simulink model "Prediction_3sAdvance_2output"  (R2016b)
settings: Solver=FixedStepAuto  StartTime=0.0  StopTime=length(lat_y)  FixedStep=1  RelTol=1e-3
StopFcn:
  | %%
  | scrsz = get(groot,'ScreenSize');
  | figure('Position',[40 scrsz(4)*0.1 scrsz(3)*0.8 scrsz(4)*0.8])
  | 
  | lng_margin = (max(LOCATIONLongitude(indices))-min(LOCATIONLongitude(indices)))*0.01;
  | lat_margin = (max(LOCATIONLatitude(indices))-min(LOCATIONLatitude(indices)))*0.01;
  | 
  | live_plot_title = ['Pedestrian Path Neural Network Prediction' newline ...
  |     'Green Rectangle:Current Position, Cyan Rectangle:Future Position' newline ...
  |     'blue line:predicted, green line:actual path'];
  | 
  | %occupy space on google map to plot the predicted trajectory
  | annotation('textbox', [0.7 0.9 0.1 0.1],'String', live_plot_title,'EdgeColor', 'k','HorizontalAlignment', 'center','FontWeight','bold');
  | 
  | %plot for acutal pedestrian path
  | subplot(1,2,1);
  | actual_lng = LOCATIONLongitude(indices);
  | actual_lat = LOCATIONLatitude(indices);
  | plot(actual_lng,actual_lat,'g','linewidth',2); hold on;
  | plot_google_map('MapType','satellite');
  | xlim([min(actual_lng)-lng_margin max(actual_lng)+lng_margin]);
  | ylim([min(actual_lat)-lat_margin max(actual_lat)+lat_margin]);
  | title('Actual Pedestrian Path');xlabel('Longitude');ylabel('Latitude');
  | 
  | 
  | predict_y = out_x.signals.values;
  | predict_x = out_y.signals.values;
  | 
  | %convert the predicted path to the latitude and longitude
  | [predict_lat,predict_lng] = utm2ll(predict_y + x_init, predict_x + y_init,zone);
  | subplot(1,2,2);
  | title('Predicted Pedestrian Path');xlabel('Longitude');ylabel('Latitude');
  | lat_lim = [min(predict_lat) min(predict_lat) max(predict_lat) max(predict_lat)];
  | long_lim = [max(predict_lng) min(predict_lng) min(predict_lng) max(predict_lng)];
  | scatter(long_lim, lat_lim);
  | plot_google_map('MapType','satellite');
  | xlim([min(predict_lng)-lng_margin max(predict_lng)+lng_margin]);
  | ylim([min(predict_lat)-lat_margin max(predict_lat)+lat_margin]);
  | for(i=1:1:length(actual_lat))
  |     plot(actual_lng(i),actual_lat(i),'gs','MarkerSize',10);hold on;
  |     plot(predict_lng(i),predict_lat(i),'bs','MarkerSize',10);hold on;
  | 
  |     RectPosCurr = [actual_lng(i)-lng_margin*2 actual_lat(i)-lat_margin*2 lng_margin*4 lat_margin*4];
  |     RectPosFuture = [predict_lng(i)-lng_margin*2 predict_lat(i)-lat_margin*2 lng_margin*4 lat_margin*4];
  |     showCurr = rectangle('Position',RectPosCurr,'FaceColor','g','Visible','on');
  |     showFuture = rectangle('Position',RectPosFuture,'FaceColor','c','Visible','on');
  |     pause(0.01/2);
  | 
  |     set(showCurr,'Visible','off');
  |     set(showFuture,'Visible','off');
  |     pause(0.01/2);
  | end
  | 
  | 
  | save('TestData_NNPred_3s.mat','indices','LOCATIONLatitude','LOCATIONLongitude','predict_lat','predict_lng');
values from neighbouring files (symbols this model uses):
  indices = [20 21 22 23 24 25 26 27 28 29 30 31 ... (1110 elements, 1110x1)]    [Circle.mat]    (also in DoubleEllipse.mat = [57 58 59 60 61 62 63 64 65 66 67 68 ... (2382 elements, 238; GPS_Path_Prediction.m = find(~isempty(orientation_temp)&~isnan(orientation_temp)); Rectangle.mat = [51 52 53 54 55 56 57 58 59 60 61 62 ... (1700 elements, 170; special_filter.m = find(variance<=var_threshold & abs(magnitude) <= mag_thresho)
  LOCATIONLatitude = [42.32249 42.32249 42.32249 42.32249 42.32249 42.32249 42.32249 42.32249 42.32249 42.32249 42.32249 42.32249 ... (1135 elements, 1135x1)]    [Circle.mat]    (also in DoubleEllipse.mat = [42.322384 42.322384 42.322384 42.322384 42.322384 42.322384; Rectangle.mat = [42.323025 42.323025 42.323025 42.323025 42.323025 42.323025)
  LOCATIONLongitude = [-83.479965 -83.479965 -83.479965 -83.479965 -83.479965 -83.479965 -83.479965 -83.479965 -83.479965 -83.479965 -83.479965 -83.479965 ... (1135 elements, 1135x1)]    [Circle.mat]    (also in DoubleEllipse.mat = [-83.47919 -83.47919 -83.47919 -83.47919 -83.47919 -83.47919; Rectangle.mat = [-83.47979 -83.47979 -83.47979 -83.47979 -83.47979 -83.47979)
libraries: neural x17
(part 1 of 2)
settings Model: Creator=divye  LastModifiedBy=divye

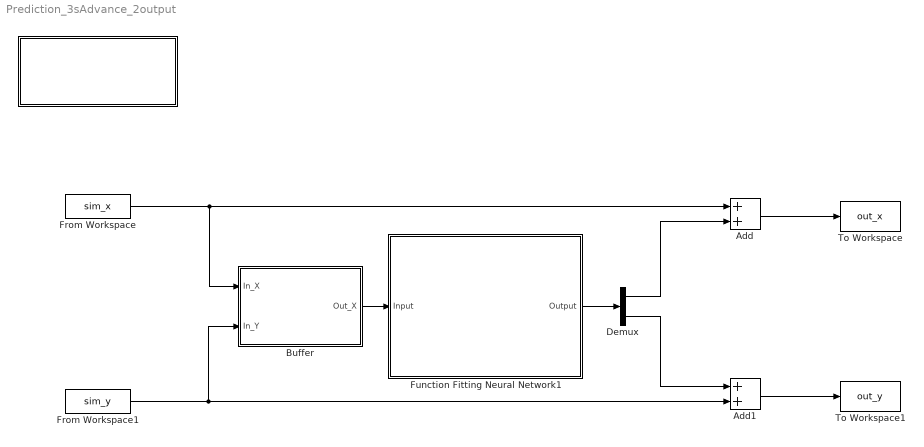
== system Prediction_3sAdvance_2output ==
  " " : Subsystem
      settings: OpenFcn=|
      | %%
      | %receive the user input for the measurement file
      | clear all;close all; %#ok<CLALL>
      | [measurement_file, measurement_file_path] = uigetfile({'*.mat'},'Measurement File Selector');
      | filename = strcat(measurement_file_path,measurement_file);
      | load(filename);
      | t=0:1:length(lng_x)-1;
      | sim_x = [t' lng_x];
      | sim_y = [t' lat_y];
      mask Display: disp(['Import' newline 'Data Set'])
  Add : Sum
  Add1 : Sum
  Buffer : Subsystem
  Demux : Demux  Outputs=2
  From Workspace : FromWorkspace  VariableName=sim_x  SampleTime=1
  From Workspace1 : FromWorkspace  VariableName=sim_y  SampleTime=1
  Function Fitting Neural Network1 : Subsystem
      mask help: Function Fitting Neural Network
      mask Display: e = 0.06;c1 = [120 150 230]/255;c2 = ([120 150 230]+0)/383;c3 = ([120 150 230]+128)/383;patch([0 1 1 0],[0 0 1 1],c1);patch([0 1 1 1-e 1-e 0+e],[0 0 1 1-e 0+e 0+e],c2);patch([0 0 1 1-e 0+e 0+e],[0 1 1 1-e 1-e 0+e],c3);plot([0 1 1 0 0],[0 0 1 1 0]);fprintf('NNET');port_label('input',1,' Input');port_label('output',1,'Output ');
  To Workspace : ToWorkspace  VariableName=out_x  SaveFormat=Structure With Time  SampleTime=-1
  To Workspace1 : ToWorkspace  VariableName=out_y  SaveFormat=Structure With Time  SampleTime=-1
  wires:
  Buffer/1(Out_X) -> Function Fitting Neural Network1/1(Input)
  Function Fitting Neural Network1/1(Output) -> Demux/1
  From Workspace/1 -> Buffer/1(In_X), Add/1
  Demux/1 -> Add/2
  Add/1 -> To Workspace/1
  Demux/2 -> Add1/1
  From Workspace1/1 -> Buffer/2(In_Y), Add1/2
  Add1/1 -> To Workspace1/1

== system Prediction_3sAdvance_2output/  ==

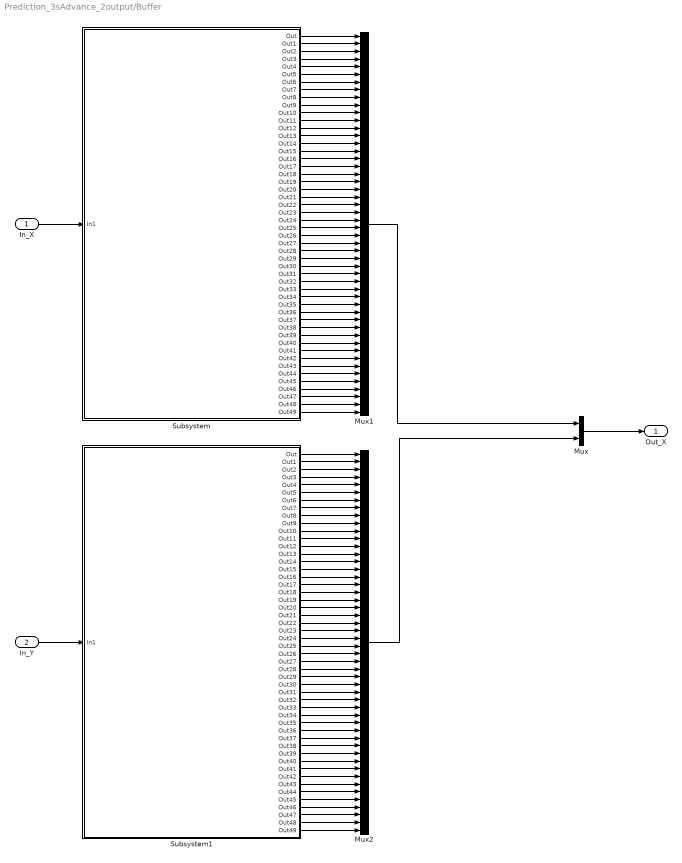
== system Prediction_3sAdvance_2output/Buffer ==
  In_X : Inport
  In_Y : Inport  Port=2
  Mux : Mux  Inputs=2
  Mux1 : Mux  Inputs=50
  Mux2 : Mux  Inputs=50
  Subsystem : Subsystem
  Subsystem1 : Subsystem
  Out_X : Outport
  wires:
  Mux1/1 -> Mux/1
  Subsystem1/46(Out45) -> Mux2/46
  Subsystem1/20(Out19) -> Mux2/20
  Subsystem1/38(Out37) -> Mux2/38
  Subsystem1/21(Out20) -> Mux2/21
  Subsystem1/42(Out41) -> Mux2/42
  Subsystem1/47(Out46) -> Mux2/47
  Subsystem1/22(Out21) -> Mux2/22
  Subsystem1/5(Out4) -> Mux2/5
  In_Y/1 -> Subsystem1/1(In1)
  Subsystem1/43(Out42) -> Mux2/43
  Subsystem1/11(Out10) -> Mux2/11
  In_X/1 -> Subsystem/1(In1)
  Subsystem1/19(Out18) -> Mux2/19
  Subsystem1/23(Out22) -> Mux2/23
  Subsystem1/17(Out16) -> Mux2/17
  Subsystem1/1(Out) -> Mux2/1
  Subsystem1/25(Out24) -> Mux2/25
  Subsystem1/44(Out43) -> Mux2/44
  Subsystem1/37(Out36) -> Mux2/37
  Subsystem1/39(Out38) -> Mux2/39
  Mux2/1 -> Mux/2
  Subsystem1/45(Out44) -> Mux2/45
  Subsystem1/41(Out40) -> Mux2/41
  Subsystem1/14(Out13) -> Mux2/14
  Subsystem1/24(Out23) -> Mux2/24
  Subsystem1/40(Out39) -> Mux2/40
  Subsystem/28(Out27) -> Mux1/28
  Subsystem/48(Out47) -> Mux1/48
  Subsystem/29(Out28) -> Mux1/29
  Subsystem/27(Out26) -> Mux1/27
  Subsystem/34(Out33) -> Mux1/34
  Subsystem/32(Out31) -> Mux1/32
  Subsystem/33(Out32) -> Mux1/33
  Subsystem/30(Out29) -> Mux1/30
  Subsystem/36(Out35) -> Mux1/36
  Subsystem/26(Out25) -> Mux1/26
  Subsystem/49(Out48) -> Mux1/49
  Subsystem/50(Out49) -> Mux1/50
  Subsystem/31(Out30) -> Mux1/31
  Subsystem/3(Out2) -> Mux1/3
  Subsystem/35(Out34) -> Mux1/35
  Subsystem/2(Out1) -> Mux1/2
  Subsystem/22(Out21) -> Mux1/22
  Subsystem/15(Out14) -> Mux1/15
  Subsystem/19(Out18) -> Mux1/19
  Subsystem/24(Out23) -> Mux1/24
  Subsystem/20(Out19) -> Mux1/20
  Subsystem/4(Out3) -> Mux1/4
  Subsystem/9(Out8) -> Mux1/9
  Subsystem/13(Out12) -> Mux1/13
  Subsystem/12(Out11) -> Mux1/12
  Subsystem/10(Out9) -> Mux1/10
  Subsystem/16(Out15) -> Mux1/16
  Subsystem/6(Out5) -> Mux1/6
  Subsystem/7(Out6) -> Mux1/7
  Subsystem/8(Out7) -> Mux1/8
  Subsystem/18(Out17) -> Mux1/18
  Subsystem/17(Out16) -> Mux1/17
  Subsystem/25(Out24) -> Mux1/25
  Subsystem/23(Out22) -> Mux1/23
  Subsystem/21(Out20) -> Mux1/21
  Subsystem/14(Out13) -> Mux1/14
  Subsystem/43(Out42) -> Mux1/43
  Subsystem/42(Out41) -> Mux1/42
  Subsystem/41(Out40) -> Mux1/41
  Subsystem/46(Out45) -> Mux1/46
  Subsystem/37(Out36) -> Mux1/37
  Subsystem/45(Out44) -> Mux1/45
  Subsystem/40(Out39) -> Mux1/40
  Subsystem/47(Out46) -> Mux1/47
  Subsystem/5(Out4) -> Mux1/5
  Subsystem/44(Out43) -> Mux1/44
  Subsystem/38(Out37) -> Mux1/38
  Subsystem/39(Out38) -> Mux1/39
  Subsystem/11(Out10) -> Mux1/11
  Subsystem/1(Out) -> Mux1/1
  Subsystem1/49(Out48) -> Mux2/49
  Subsystem1/48(Out47) -> Mux2/48
  Subsystem1/50(Out49) -> Mux2/50
  Subsystem1/28(Out27) -> Mux2/28
  Subsystem1/29(Out28) -> Mux2/29
  Subsystem1/33(Out32) -> Mux2/33
  Subsystem1/4(Out3) -> Mux2/4
  Subsystem1/2(Out1) -> Mux2/2
  Subsystem1/9(Out8) -> Mux2/9
  Subsystem1/30(Out29) -> Mux2/30
  Subsystem1/31(Out30) -> Mux2/31
  Subsystem1/34(Out33) -> Mux2/34
  Subsystem1/32(Out31) -> Mux2/32
  Subsystem1/13(Out12) -> Mux2/13
  Subsystem1/10(Out9) -> Mux2/10
  Subsystem1/15(Out14) -> Mux2/15
  Subsystem1/26(Out25) -> Mux2/26
  Subsystem1/27(Out26) -> Mux2/27
  Subsystem1/8(Out7) -> Mux2/8
  Subsystem1/18(Out17) -> Mux2/18
  Subsystem1/16(Out15) -> Mux2/16
  Subsystem1/36(Out35) -> Mux2/36
  Subsystem1/12(Out11) -> Mux2/12
  Subsystem1/35(Out34) -> Mux2/35
  Subsystem1/7(Out6) -> Mux2/7
  Subsystem1/3(Out2) -> Mux2/3
  Subsystem1/6(Out5) -> Mux2/6
  Mux/1 -> Out_X/1

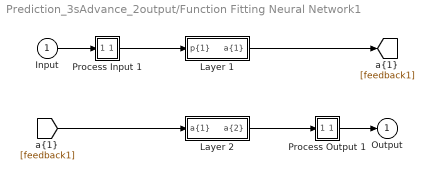
== system Prediction_3sAdvance_2output/Function Fitting Neural Network1 ==
  Input : Inport  PortDimensions=100
      mask Display: e = 0.06;c1 = [120 230 180]/255;c2 = ([120 230 180]+0)/(256+128);c3 = ([120 230 180]+128)/(256+128);patch([0 1 1 0],[0 0 1 1],c1);patch([0 1 1 1-e 1-e 0+e],[0 0 1 1-e 0+e 0+e],c2);patch([0 0 1 1-e 0+e 0+e],[0 1 1 1-e 1-e 0+e],c3);plot([0 1 1 0 0],[0 0 1 1 0]);
  Layer 1 : Subsystem
      mask Display: e = 0.06;c1 = [120 150 230]/255;c2 = ([120 150 230]+0)/383;c3 = ([120 150 230]+128)/383;patch([0 1 1 0],[0 0 1 1],c1);patch([0 1 1 1-e 1-e 0+e],[0 0 1 1-e 0+e 0+e],c2);patch([0 0 1 1-e 0+e 0+e],[0 1 1 1-e 1-e 0+e],c3);plot([0 1 1 0 0],[0 0 1 1 0]);
  Layer 2 : Subsystem
      mask Display: e = 0.06;c1 = [120 150 230]/255;c2 = ([120 150 230]+0)/383;c3 = ([120 150 230]+128)/383;patch([0 1 1 0],[0 0 1 1],c1);patch([0 1 1 1-e 1-e 0+e],[0 0 1 1-e 0+e 0+e],c2);patch([0 0 1 1-e 0+e 0+e],[0 1 1 1-e 1-e 0+e],c3);plot([0 1 1 0 0],[0 0 1 1 0]);
  Process Input 1 : Subsystem
      mask Display: e = 0.06;c1 = [120 150 230]/255;c2 = ([120 150 230]+0)/383;c3 = ([120 150 230]+128)/383;patch([0 1 1 0],[0 0 1 1],c1);patch([0 1 1 1-e 1-e 0+e],[0 0 1 1-e 0+e 0+e],c2);patch([0 0 1 1-e 0+e 0+e],[0 1 1 1-e 1-e 0+e],c3);plot([0 1 1 0 0],[0 0 1 1 0]);
  Process Output 1 : Subsystem
      mask Display: e = 0.06;c1 = [120 150 230]/255;c2 = ([120 150 230]+0)/383;c3 = ([120 150 230]+128)/383;patch([0 1 1 0],[0 0 1 1],c1);patch([0 1 1 1-e 1-e 0+e],[0 0 1 1-e 0+e 0+e],c2);patch([0 0 1 1-e 0+e 0+e],[0 1 1 1-e 1-e 0+e],c3);plot([0 1 1 0 0],[0 0 1 1 0]);
  Output : Outport  InitialOutput=[0;0]
      mask Display: e = 0.06;c1 = [120 230 180]/255;c2 = ([120 230 180]+0)/(256+128);c3 = ([120 230 180]+128)/(256+128);patch([0 1 1 0],[0 0 1 1],c1);patch([0 1 1 1-e 1-e 0+e],[0 0 1 1-e 0+e 0+e],c2);patch([0 0 1 1-e 0+e 0+e],[0 1 1 1-e 1-e 0+e],c3);plot([0 1 1 0 0],[0 0 1 1 0]);
  wires:
  Input/1 -> Process Input 1/1(x)
  Process Output 1/1(y) -> Output/1
  Process Input 1/1(p) -> Layer 1/1("p{1}")
  Layer 1/1("a{1}") -> [feedback1]
  [feedback1] -> Layer 2/1("a{1} ")
  Layer 2/1("a{2}") -> Process Output 1/1(a)

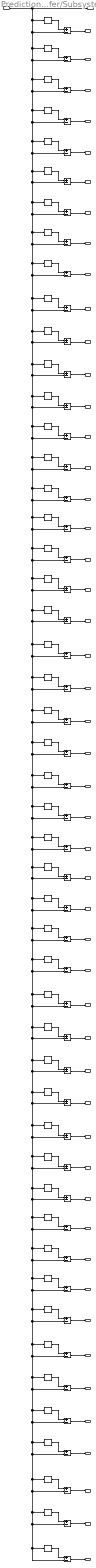
== system Prediction_3sAdvance_2output/Buffer/Subsystem ==
  In1 : Inport
  Delay : Delay  DelayLength=1
  Delay1 : Delay
  Delay10 : Delay  DelayLength=11
  Delay11 : Delay  DelayLength=12
  Delay12 : Delay  DelayLength=13
  Delay13 : Delay  DelayLength=22
  Delay14 : Delay  DelayLength=23
  Delay15 : Delay  DelayLength=24
  Delay16 : Delay  DelayLength=14
  Delay17 : Delay  DelayLength=15
  Delay18 : Delay  DelayLength=16
  Delay19 : Delay  DelayLength=17
  Delay2 : Delay  DelayLength=3
  Delay20 : Delay  DelayLength=18
  Delay21 : Delay  DelayLength=19
  Delay22 : Delay  DelayLength=20
  Delay23 : Delay  DelayLength=21
  Delay24 : Delay  DelayLength=33
  Delay25 : Delay  DelayLength=34
  Delay26 : Delay  DelayLength=35
  Delay27 : Delay  DelayLength=25
  Delay28 : Delay  DelayLength=26
  Delay29 : Delay  DelayLength=27
  Delay3 : Delay  DelayLength=4
  Delay30 : Delay  DelayLength=28
  Delay31 : Delay  DelayLength=29
  Delay32 : Delay  DelayLength=30
  Delay33 : Delay  DelayLength=31
  Delay34 : Delay  DelayLength=32
  Delay35 : Delay  DelayLength=44
  Delay36 : Delay  DelayLength=45
  Delay37 : Delay  DelayLength=46
  Delay38 : Delay  DelayLength=36
  Delay39 : Delay  DelayLength=37
  Delay4 : Delay  DelayLength=5
  Delay40 : Delay  DelayLength=38
  Delay41 : Delay  DelayLength=39
  Delay42 : Delay  DelayLength=40
  Delay43 : Delay  DelayLength=41
  Delay44 : Delay  DelayLength=42
  Delay45 : Delay  DelayLength=43
  Delay46 : Delay  DelayLength=47
  Delay47 : Delay  DelayLength=48
  Delay48 : Delay  DelayLength=49
  Delay5 : Delay  DelayLength=6
  Delay6 : Delay  DelayLength=7
  Delay7 : Delay  DelayLength=8
  Delay8 : Delay  DelayLength=9
  Delay9 : Delay  DelayLength=10
  Subtract{,1..48} (49 alike) : Sum  Inputs=+-
  Out : Outport
  Out1 : Outport  Port=2
  Out2 : Outport  Port=3
  Out3 : Outport  Port=4
  Out4 : Outport  Port=5
  Out5 : Outport  Port=6
  Out6 : Outport  Port=7
  Out7 : Outport  Port=8
  Out8 : Outport  Port=9
  Out9 : Outport  Port=10
  Out10 : Outport  Port=11
  Out11 : Outport  Port=12
  Out12 : Outport  Port=13
  Out13 : Outport  Port=14
  Out14 : Outport  Port=15
  Out15 : Outport  Port=16
  Out16 : Outport  Port=17
  Out17 : Outport  Port=18
  Out18 : Outport  Port=19
  Out19 : Outport  Port=20
  Out20 : Outport  Port=21
  Out21 : Outport  Port=22
  Out22 : Outport  Port=23
  Out23 : Outport  Port=24
  Out24 : Outport  Port=25
  Out25 : Outport  Port=26
  Out26 : Outport  Port=27
  Out27 : Outport  Port=28
  Out28 : Outport  Port=29
  Out29 : Outport  Port=30
  Out30 : Outport  Port=31
  Out31 : Outport  Port=32
  Out32 : Outport  Port=33
  Out33 : Outport  Port=34
  Out34 : Outport  Port=35
  Out35 : Outport  Port=36
  Out36 : Outport  Port=37
  Out37 : Outport  Port=38
  Out38 : Outport  Port=39
  Out39 : Outport  Port=40
  Out40 : Outport  Port=41
  Out41 : Outport  Port=42
  Out42 : Outport  Port=43
  Out43 : Outport  Port=44
  Out44 : Outport  Port=45
  Out45 : Outport  Port=46
  Out46 : Outport  Port=47
  Out47 : Outport  Port=48
  Out48 : Outport  Port=49
  Out49 : Outport  Port=50
  wires:
  Delay/1 -> Subtract/1
  Subtract/1 -> Out1/1
  Delay1/1 -> Subtract1/1
  Subtract1/1 -> Out2/1
  Delay2/1 -> Subtract2/1
  Subtract2/1 -> Out3/1
  Delay3/1 -> Subtract3/1
  Subtract3/1 -> Out4/1
  Delay4/1 -> Subtract4/1
  Subtract4/1 -> Out5/1
  Delay5/1 -> Subtract5/1
  Subtract5/1 -> Out6/1
  Delay6/1 -> Subtract6/1
  Subtract6/1 -> Out7/1
  Delay7/1 -> Subtract7/1
  Subtract7/1 -> Out8/1
  Delay8/1 -> Subtract8/1
  Subtract8/1 -> Out9/1
  Delay9/1 -> Subtract9/1
  Subtract9/1 -> Out10/1
  Delay10/1 -> Subtract10/1
  Subtract10/1 -> Out11/1
  Delay11/1 -> Subtract11/1
  Subtract11/1 -> Out12/1
  Delay12/1 -> Subtract12/1
  Subtract12/1 -> Out13/1
  Delay16/1 -> Subtract16/1
  Subtract16/1 -> Out14/1
  Delay17/1 -> Subtract17/1
  Subtract17/1 -> Out15/1
  Delay18/1 -> Subtract18/1
  Subtract18/1 -> Out16/1
  Delay19/1 -> Subtract19/1
  Subtract19/1 -> Out17/1
  Delay20/1 -> Subtract20/1
  Subtract20/1 -> Out18/1
  Delay21/1 -> Subtract21/1
  Subtract21/1 -> Out19/1
  Delay22/1 -> Subtract22/1
  Subtract22/1 -> Out20/1
  Delay23/1 -> Subtract23/1
  Subtract23/1 -> Out21/1
  Delay13/1 -> Subtract13/1
  Subtract13/1 -> Out22/1
  Delay14/1 -> Subtract14/1
  Subtract14/1 -> Out23/1
  Delay15/1 -> Subtract15/1
  Subtract15/1 -> Out24/1
  Delay27/1 -> Subtract27/1
  Subtract27/1 -> Out25/1
  Delay28/1 -> Subtract28/1
  Subtract28/1 -> Out26/1
  Delay29/1 -> Subtract29/1
  Subtract29/1 -> Out27/1
  Delay30/1 -> Subtract30/1
  Subtract30/1 -> Out28/1
  Delay31/1 -> Subtract31/1
  Subtract31/1 -> Out29/1
  Delay32/1 -> Subtract32/1
  Subtract32/1 -> Out30/1
  Delay33/1 -> Subtract33/1
  Subtract33/1 -> Out31/1
  Delay34/1 -> Subtract34/1
  Subtract34/1 -> Out32/1
  Delay24/1 -> Subtract24/1
  Subtract24/1 -> Out33/1
  Delay25/1 -> Subtract25/1
  Subtract25/1 -> Out34/1
  Delay26/1 -> Subtract26/1
  Subtract26/1 -> Out35/1
  Delay38/1 -> Subtract38/1
  Subtract38/1 -> Out36/1
  Delay39/1 -> Subtract39/1
  Subtract39/1 -> Out37/1
  Delay40/1 -> Subtract40/1
  Subtract40/1 -> Out38/1
  Delay41/1 -> Subtract41/1
  Subtract41/1 -> Out39/1
  Delay42/1 -> Subtract42/1
  Subtract42/1 -> Out40/1
  Delay43/1 -> Subtract43/1
  Subtract43/1 -> Out41/1
  Delay44/1 -> Subtract44/1
  Subtract44/1 -> Out42/1
  Delay45/1 -> Subtract45/1
  Subtract45/1 -> Out43/1
  Delay35/1 -> Subtract35/1
  Subtract35/1 -> Out44/1
  Delay36/1 -> Subtract36/1
  Subtract36/1 -> Out45/1
  Delay37/1 -> Subtract37/1
  Subtract37/1 -> Out46/1
  Delay46/1 -> Subtract46/1
  Subtract46/1 -> Out47/1
  Delay47/1 -> Subtract47/1
  Subtract47/1 -> Out48/1
  Delay48/1 -> Subtract48/1
  Subtract48/1 -> Out49/1
  In1/1 -> Out/1, Delay/1, Subtract/2, Delay1/1, Delay2/1, Delay3/1, Delay4/1, Delay5/1, Delay6/1, Delay7/1, Delay8/1, Delay9/1, Delay10/1, Delay11/1, Delay12/1, Delay16/1, Delay17/1, Delay18/1, Delay19/1, Delay20/1, Delay21/1, Delay22/1, Delay23/1, Delay13/1, Delay14/1, Delay15/1, Delay27/1, Delay28/1, Delay29/1, Delay30/1, Delay31/1, Delay32/1, Delay33/1, Delay34/1, Delay24/1, Delay25/1, Delay26/1, Delay38/1, Delay39/1, Delay40/1, Delay41/1, Delay42/1, Delay43/1, Delay44/1, Delay45/1, Delay35/1, Delay36/1, Delay37/1, Delay46/1, Delay47/1, Delay48/1, Subtract48/2, Subtract47/2, Subtract46/2, Subtract37/2, Subtract36/2, Subtract35/2, Subtract45/2, Subtract44/2, Subtract43/2, Subtract42/2, Subtract41/2, Subtract40/2, Subtract39/2, Subtract38/2, Subtract26/2, Subtract25/2, Subtract24/2, Subtract34/2, Subtract33/2, Subtract32/2, Subtract31/2, Subtract30/2, Subtract29/2, Subtract28/2, Subtract27/2, Subtract15/2, Subtract14/2, Subtract13/2, Subtract23/2, Subtract22/2, Subtract21/2, Subtract20/2, Subtract19/2, Subtract18/2, Subtract17/2, Subtract16/2, Subtract12/2, Subtract11/2, Subtract10/2, Subtract9/2, Subtract8/2, Subtract7/2, Subtract6/2, Subtract5/2, Subtract4/2, Subtract3/2, Subtract2/2, Subtract1/2

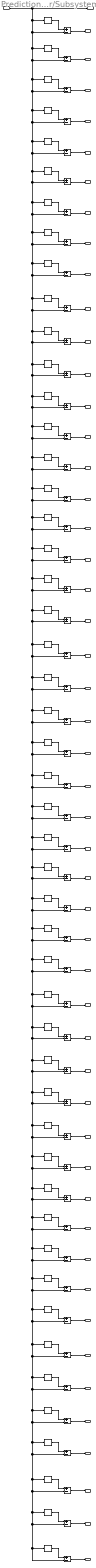
== system Prediction_3sAdvance_2output/Buffer/Subsystem1 ==
  In1 : Inport
  Delay : Delay  DelayLength=1
  Delay1 : Delay
  Delay10 : Delay  DelayLength=11
  Delay11 : Delay  DelayLength=12
  Delay12 : Delay  DelayLength=13
  Delay13 : Delay  DelayLength=22
  Delay14 : Delay  DelayLength=23
  Delay15 : Delay  DelayLength=24
  Delay16 : Delay  DelayLength=14
  Delay17 : Delay  DelayLength=15
  Delay18 : Delay  DelayLength=16
  Delay19 : Delay  DelayLength=17
  Delay2 : Delay  DelayLength=3
  Delay20 : Delay  DelayLength=18
  Delay21 : Delay  DelayLength=19
  Delay22 : Delay  DelayLength=20
  Delay23 : Delay  DelayLength=21
  Delay24 : Delay  DelayLength=33
  Delay25 : Delay  DelayLength=34
  Delay26 : Delay  DelayLength=35
  Delay27 : Delay  DelayLength=25
  Delay28 : Delay  DelayLength=26
  Delay29 : Delay  DelayLength=27
  Delay3 : Delay  DelayLength=4
  Delay30 : Delay  DelayLength=28
  Delay31 : Delay  DelayLength=29
  Delay32 : Delay  DelayLength=30
  Delay33 : Delay  DelayLength=31
  Delay34 : Delay  DelayLength=32
  Delay35 : Delay  DelayLength=44
  Delay36 : Delay  DelayLength=45
  Delay37 : Delay  DelayLength=46
  Delay38 : Delay  DelayLength=36
  Delay39 : Delay  DelayLength=37
  Delay4 : Delay  DelayLength=5
  Delay40 : Delay  DelayLength=38
  Delay41 : Delay  DelayLength=39
  Delay42 : Delay  DelayLength=40
  Delay43 : Delay  DelayLength=41
  Delay44 : Delay  DelayLength=42
  Delay45 : Delay  DelayLength=43
  Delay46 : Delay  DelayLength=47
  Delay47 : Delay  DelayLength=48
  Delay48 : Delay  DelayLength=49
  Delay5 : Delay  DelayLength=6
  Delay6 : Delay  DelayLength=7
  Delay7 : Delay  DelayLength=8
  Delay8 : Delay  DelayLength=9
  Delay9 : Delay  DelayLength=10
  Subtract{,1..48} (49 alike) : Sum  Inputs=+-
  Out : Outport
  Out1 : Outport  Port=2
  Out2 : Outport  Port=3
  Out3 : Outport  Port=4
  Out4 : Outport  Port=5
  Out5 : Outport  Port=6
  Out6 : Outport  Port=7
  Out7 : Outport  Port=8
  Out8 : Outport  Port=9
  Out9 : Outport  Port=10
  Out10 : Outport  Port=11
  Out11 : Outport  Port=12
  Out12 : Outport  Port=13
  Out13 : Outport  Port=14
  Out14 : Outport  Port=15
  Out15 : Outport  Port=16
  Out16 : Outport  Port=17
  Out17 : Outport  Port=18
  Out18 : Outport  Port=19
  Out19 : Outport  Port=20
  Out20 : Outport  Port=21
  Out21 : Outport  Port=22
  Out22 : Outport  Port=23
  Out23 : Outport  Port=24
  Out24 : Outport  Port=25
  Out25 : Outport  Port=26
  Out26 : Outport  Port=27
  Out27 : Outport  Port=28
  Out28 : Outport  Port=29
  Out29 : Outport  Port=30
  Out30 : Outport  Port=31
  Out31 : Outport  Port=32
  Out32 : Outport  Port=33
  Out33 : Outport  Port=34
  Out34 : Outport  Port=35
  Out35 : Outport  Port=36
  Out36 : Outport  Port=37
  Out37 : Outport  Port=38
  Out38 : Outport  Port=39
  Out39 : Outport  Port=40
  Out40 : Outport  Port=41
  Out41 : Outport  Port=42
  Out42 : Outport  Port=43
  Out43 : Outport  Port=44
  Out44 : Outport  Port=45
  Out45 : Outport  Port=46
  Out46 : Outport  Port=47
  Out47 : Outport  Port=48
  Out48 : Outport  Port=49
  Out49 : Outport  Port=50
  wires:
  Delay/1 -> Subtract/1
  Subtract/1 -> Out1/1
  Delay1/1 -> Subtract1/1
  Subtract1/1 -> Out2/1
  Delay2/1 -> Subtract2/1
  Subtract2/1 -> Out3/1
  Delay3/1 -> Subtract3/1
  Subtract3/1 -> Out4/1
  Delay4/1 -> Subtract4/1
  Subtract4/1 -> Out5/1
  Delay5/1 -> Subtract5/1
  Subtract5/1 -> Out6/1
  Delay6/1 -> Subtract6/1
  Subtract6/1 -> Out7/1
  Delay7/1 -> Subtract7/1
  Subtract7/1 -> Out8/1
  Delay8/1 -> Subtract8/1
  Subtract8/1 -> Out9/1
  Delay9/1 -> Subtract9/1
  Subtract9/1 -> Out10/1
  Delay10/1 -> Subtract10/1
  Subtract10/1 -> Out11/1
  Delay11/1 -> Subtract11/1
  Subtract11/1 -> Out12/1
  Delay12/1 -> Subtract12/1
  Subtract12/1 -> Out13/1
  Delay16/1 -> Subtract16/1
  Subtract16/1 -> Out14/1
  Delay17/1 -> Subtract17/1
  Subtract17/1 -> Out15/1
  Delay18/1 -> Subtract18/1
  Subtract18/1 -> Out16/1
  Delay19/1 -> Subtract19/1
  Subtract19/1 -> Out17/1
  Delay20/1 -> Subtract20/1
  Subtract20/1 -> Out18/1
  Delay21/1 -> Subtract21/1
  Subtract21/1 -> Out19/1
  Delay22/1 -> Subtract22/1
  Subtract22/1 -> Out20/1
  Delay23/1 -> Subtract23/1
  Subtract23/1 -> Out21/1
  Delay13/1 -> Subtract13/1
  Subtract13/1 -> Out22/1
  Delay14/1 -> Subtract14/1
  Subtract14/1 -> Out23/1
  Delay15/1 -> Subtract15/1
  Subtract15/1 -> Out24/1
  Delay27/1 -> Subtract27/1
  Subtract27/1 -> Out25/1
  Delay28/1 -> Subtract28/1
  Subtract28/1 -> Out26/1
  Delay29/1 -> Subtract29/1
  Subtract29/1 -> Out27/1
  Delay30/1 -> Subtract30/1
  Subtract30/1 -> Out28/1
  Delay31/1 -> Subtract31/1
  Subtract31/1 -> Out29/1
  Delay32/1 -> Subtract32/1
  Subtract32/1 -> Out30/1
  Delay33/1 -> Subtract33/1
  Subtract33/1 -> Out31/1
  Delay34/1 -> Subtract34/1
  Subtract34/1 -> Out32/1
  Delay24/1 -> Subtract24/1
  Subtract24/1 -> Out33/1
  Delay25/1 -> Subtract25/1
  Subtract25/1 -> Out34/1
  Delay26/1 -> Subtract26/1
  Subtract26/1 -> Out35/1
  Delay38/1 -> Subtract38/1
  Subtract38/1 -> Out36/1
  Delay39/1 -> Subtract39/1
  Subtract39/1 -> Out37/1
  Delay40/1 -> Subtract40/1
  Subtract40/1 -> Out38/1
  Delay41/1 -> Subtract41/1
  Subtract41/1 -> Out39/1
  Delay42/1 -> Subtract42/1
  Subtract42/1 -> Out40/1
  Delay43/1 -> Subtract43/1
  Subtract43/1 -> Out41/1
  Delay44/1 -> Subtract44/1
  Subtract44/1 -> Out42/1
  Delay45/1 -> Subtract45/1
  Subtract45/1 -> Out43/1
  Delay35/1 -> Subtract35/1
  Subtract35/1 -> Out44/1
  Delay36/1 -> Subtract36/1
  Subtract36/1 -> Out45/1
  Delay37/1 -> Subtract37/1
  Subtract37/1 -> Out46/1
  Delay46/1 -> Subtract46/1
  Subtract46/1 -> Out47/1
  Delay47/1 -> Subtract47/1
  Subtract47/1 -> Out48/1
  Delay48/1 -> Subtract48/1
  Subtract48/1 -> Out49/1
  In1/1 -> Out/1, Delay/1, Subtract/2, Delay1/1, Delay2/1, Delay3/1, Delay4/1, Delay5/1, Delay6/1, Delay7/1, Delay8/1, Delay9/1, Delay10/1, Delay11/1, Delay12/1, Delay16/1, Delay17/1, Delay18/1, Delay19/1, Delay20/1, Delay21/1, Delay22/1, Delay23/1, Delay13/1, Delay14/1, Delay15/1, Delay27/1, Delay28/1, Delay29/1, Delay30/1, Delay31/1, Delay32/1, Delay33/1, Delay34/1, Delay24/1, Delay25/1, Delay26/1, Delay38/1, Delay39/1, Delay40/1, Delay41/1, Delay42/1, Delay43/1, Delay44/1, Delay45/1, Delay35/1, Delay36/1, Delay37/1, Delay46/1, Delay47/1, Delay48/1, Subtract48/2, Subtract47/2, Subtract46/2, Subtract37/2, Subtract36/2, Subtract35/2, Subtract45/2, Subtract44/2, Subtract43/2, Subtract42/2, Subtract41/2, Subtract40/2, Subtract39/2, Subtract38/2, Subtract26/2, Subtract25/2, Subtract24/2, Subtract34/2, Subtract33/2, Subtract32/2, Subtract31/2, Subtract30/2, Subtract29/2, Subtract28/2, Subtract27/2, Subtract15/2, Subtract14/2, Subtract13/2, Subtract23/2, Subtract22/2, Subtract21/2, Subtract20/2, Subtract19/2, Subtract18/2, Subtract17/2, Subtract16/2, Subtract12/2, Subtract11/2, Subtract10/2, Subtract9/2, Subtract8/2, Subtract7/2, Subtract6/2, Subtract5/2, Subtract4/2, Subtract3/2, Subtract2/2, Subtract1/2

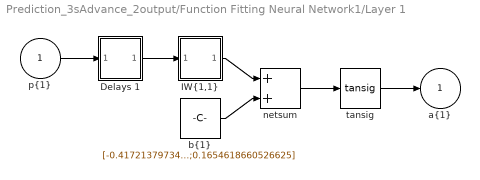
== system Prediction_3sAdvance_2output/Function Fitting Neural Network1/Layer 1 ==
  "p{1}" : Inport  PortDimensions=98
      mask Display: e = 0.06;c1 = [120 230 180]/255;c2 = ([120 230 180]+0)/(256+128);c3 = ([120 230 180]+128)/(256+128);patch([0 1 1 0],[0 0 1 1],c1);patch([0 1 1 1-e 1-e 0+e],[0 0 1 1-e 0+e 0+e],c2);patch([0 0 1 1-e 0+e 0+e],[0 1 1 1-e 1-e 0+e],c3);plot([0 1 1 0 0],[0 0 1 1 0]);
  Delays 1 : Subsystem
      mask Display: e = 0.06;c1 = [120 150 230]/255;c2 = ([120 150 230]+0)/383;c3 = ([120 150 230]+128)/383;patch([0 1 1 0],[0 0 1 1],c1);patch([0 1 1 1-e 1-e 0+e],[0 0 1 1-e 0+e 0+e],c2);patch([0 0 1 1-e 0+e 0+e],[0 1 1 1-e 1-e 0+e],c3);plot([0 1 1 0 0],[0 0 1 1 0]);disp('0');
  "IW{1,1}" : Subsystem
      mask Display: e = 0.06;c1 = [120 150 230]/255;c2 = ([120 150 230]+0)/383;c3 = ([120 150 230]+128)/383;patch([0 1 1 0],[0 0 1 1],c1);patch([0 1 1 1-e 1-e 0+e],[0 0 1 1-e 0+e 0+e],c2);patch([0 0 1 1-e 0+e 0+e],[0 1 1 1-e 1-e 0+e],c3);plot([0 1 1 0 0],[0 0 1 1 0]);disp('W');
  "b{1}" : Constant  Value=[-0.41721379734681036;-0.25154480672700869;0.23985399354268783;0.30750090765798449;-0.47802697511933573;0.040020410928868169;-0.087149329135770795;0.30775217103319574;0.16446617888273593;0.1654618660526625]
      mask Display: e = 0.06;c1 = [120 150 230]/255;c2 = ([120 150 230]+0)/383;c3 = ([120 150 230]+128)/383;patch([0 1 1 0],[0 0 1 1],c1);patch([0 1 1 1-e 1-e 0+e],[0 0 1 1-e 0+e 0+e],c2);patch([0 0 1 1-e 0+e 0+e],[0 1 1 1-e 1-e 0+e],c3);plot([0 1 1 0 0],[0 0 1 1 0]);disp('b');
  netsum : Sum  Inputs=2  SaturateOnIntegerOverflow=on  InputSameDT=on  OutDataTypeStr=Inherit: Same as first input
      mask Display: e = 0.06;c1 = [120 150 230]/255;c2 = ([120 150 230]+0)/383;c3 = ([120 150 230]+128)/383;patch([0 1 1 0],[0 0 1 1],c1);patch([0 1 1 1-e 1-e 0+e],[0 0 1 1-e 0+e 0+e],c2);patch([0 0 1 1-e 0+e 0+e],[0 1 1 1-e 1-e 0+e],c3);plot([0 1 1 0 0],[0 0 1 1 0]);disp('+');
  tansig : neural/Transfer Functions/tansig
  "a{1}" : Outport  InitialOutput=[0;0;0;0;0;0;0;0;0;0]
      mask Display: e = 0.06;c1 = [120 230 180]/255;c2 = ([120 230 180]+0)/(256+128);c3 = ([120 230 180]+128)/(256+128);patch([0 1 1 0],[0 0 1 1],c1);patch([0 1 1 1-e 1-e 0+e],[0 0 1 1-e 0+e 0+e],c2);patch([0 0 1 1-e 0+e 0+e],[0 1 1 1-e 1-e 0+e],c3);plot([0 1 1 0 0],[0 0 1 1 0]);
  wires:
  "p{1}"/1 -> Delays 1/1("p{1}")
  Delays 1/1("pd{1,1}") -> "IW{1,1}"/1("pd{1,1}")
  "IW{1,1}"/1("iz{1,1}") -> netsum/1
  "b{1}"/1 -> netsum/2
  netsum/1 -> tansig/1
  tansig/1 -> "a{1}"/1

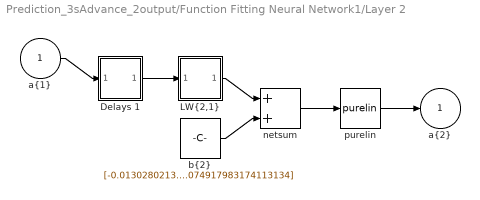
== system Prediction_3sAdvance_2output/Function Fitting Neural Network1/Layer 2 ==
  "a{1} " : Inport  PortDimensions=10
      mask Display: e = 0.06;c1 = [120 230 180]/255;c2 = ([120 230 180]+0)/(256+128);c3 = ([120 230 180]+128)/(256+128);patch([0 1 1 0],[0 0 1 1],c1);patch([0 1 1 1-e 1-e 0+e],[0 0 1 1-e 0+e 0+e],c2);patch([0 0 1 1-e 0+e 0+e],[0 1 1 1-e 1-e 0+e],c3);plot([0 1 1 0 0],[0 0 1 1 0]);
  Delays 1 : Subsystem
      mask Display: e = 0.06;c1 = [120 150 230]/255;c2 = ([120 150 230]+0)/383;c3 = ([120 150 230]+128)/383;patch([0 1 1 0],[0 0 1 1],c1);patch([0 1 1 1-e 1-e 0+e],[0 0 1 1-e 0+e 0+e],c2);patch([0 0 1 1-e 0+e 0+e],[0 1 1 1-e 1-e 0+e],c3);plot([0 1 1 0 0],[0 0 1 1 0]);disp('0');
  "LW{2,1}" : Subsystem
      mask Display: e = 0.06;c1 = [120 150 230]/255;c2 = ([120 150 230]+0)/383;c3 = ([120 150 230]+128)/383;patch([0 1 1 0],[0 0 1 1],c1);patch([0 1 1 1-e 1-e 0+e],[0 0 1 1-e 0+e 0+e],c2);patch([0 0 1 1-e 0+e 0+e],[0 1 1 1-e 1-e 0+e],c3);plot([0 1 1 0 0],[0 0 1 1 0]);disp('W');
  "b{2}" : Constant  Value=[-0.013028021350499051;-0.074917983174113134]
      mask Display: e = 0.06;c1 = [120 150 230]/255;c2 = ([120 150 230]+0)/383;c3 = ([120 150 230]+128)/383;patch([0 1 1 0],[0 0 1 1],c1);patch([0 1 1 1-e 1-e 0+e],[0 0 1 1-e 0+e 0+e],c2);patch([0 0 1 1-e 0+e 0+e],[0 1 1 1-e 1-e 0+e],c3);plot([0 1 1 0 0],[0 0 1 1 0]);disp('b');
  netsum : Sum  Inputs=2  SaturateOnIntegerOverflow=on  InputSameDT=on  OutDataTypeStr=Inherit: Same as first input
      mask Display: e = 0.06;c1 = [120 150 230]/255;c2 = ([120 150 230]+0)/383;c3 = ([120 150 230]+128)/383;patch([0 1 1 0],[0 0 1 1],c1);patch([0 1 1 1-e 1-e 0+e],[0 0 1 1-e 0+e 0+e],c2);patch([0 0 1 1-e 0+e 0+e],[0 1 1 1-e 1-e 0+e],c3);plot([0 1 1 0 0],[0 0 1 1 0]);disp('+');
  purelin : neural/Transfer Functions/purelin
  "a{2}" : Outport  InitialOutput=[0;0]
      mask Display: e = 0.06;c1 = [120 230 180]/255;c2 = ([120 230 180]+0)/(256+128);c3 = ([120 230 180]+128)/(256+128);patch([0 1 1 0],[0 0 1 1],c1);patch([0 1 1 1-e 1-e 0+e],[0 0 1 1-e 0+e 0+e],c2);patch([0 0 1 1-e 0+e 0+e],[0 1 1 1-e 1-e 0+e],c3);plot([0 1 1 0 0],[0 0 1 1 0]);
  wires:
  "a{1} "/1 -> Delays 1/1("p{2}")
  Delays 1/1("pd{2,1}") -> "LW{2,1}"/1("ad{2,1}")
  "LW{2,1}"/1("lz{2,1}") -> netsum/1
  "b{2}"/1 -> netsum/2
  netsum/1 -> purelin/1
  purelin/1 -> "a{2}"/1

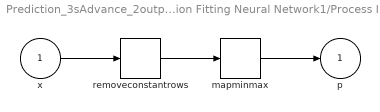
== system Prediction_3sAdvance_2output/Function Fitting Neural Network1/Process Input 1 ==
  x : Inport  PortDimensions=100
      mask Display: e = 0.06;c1 = [120 230 180]/255;c2 = ([120 230 180]+0)/(256+128);c3 = ([120 230 180]+128)/(256+128);patch([0 1 1 0],[0 0 1 1],c1);patch([0 1 1 1-e 1-e 0+e],[0 0 1 1-e 0+e 0+e],c2);patch([0 0 1 1-e 0+e 0+e],[0 1 1 1-e 1-e 0+e],c3);plot([0 1 1 0 0],[0 0 1 1 0]);
  mapminmax : neural/Processing Functions/mapminmax  xmin=[-3.2962219010223635;-3.2962219010223635;-3.2962219010223635;-3.6096502931904979;-3.6096502931904979;-3.6096502931904979;-3.6096502931904979;-3.6096502931904979;-3.6096502931904979;-4.4369455363485031;-4.9767144024372101;-4.9767144024372101;-4.9767144024372101;-5.7424785270704888;-5.7424785270704888;-5.7424785270704888;-5.7424785270704888;-5.7424785270704888;-5.7424785270704888;-6.592443810775876;-6.624825156701263;-6.624825156701263;-6.624825156701263;-6.624825156701263;-6.624825156701263;-6.624825156701263;-6.624825156701263;-6.624825156701263;-6.624825156701263;-7.8414806934306398;-9.1067063672235236;-9.1067063672235236;-9.1067063672235236;-9.1067063672235236;-9.1067063672235236;-9.1067063672235236;-9.1067063672235236;-9.1067063672235236;-9.1067063672235236;-9.3942318066838197;-9.3942318066838197;-9.9404762167250738;-9.9404762167250738;-9.9404762167250738;-9.9404762167250738;-9.9404762167250738;-9.9404762167250738;-9.9404762167250738;-9.9404762167250738;-3.6260513132438064;-3.6260513132438064;-3.6260513132438064;-3.6260513132438064;-3.6260513132438064;-3.6260513132438064;-3.8865743596106768;-3.8865743596106768;-3.9976197928190231;-5.6998751545324922;-5.6998751545324922;-5.6998751545324922;-5.6998751545324922;-5.6998751545324922;-5.6998751545324922;-5.6998751545324922;-5.6998751545324922;-5.6998751545324922;-5.6998751545324922;-5.9964295607060194;-6.9093597447499633;-6.9093597447499633;-6.9093597447499633;-6.9093597447499633;-6.9093597447499633;-8.1062844172120094;-8.1062844172120094;-8.1062844172120094;-8.1062844172120094;-8.7490837695077062;-8.7490837695077062;-8.7490837695077062;-8.7490837695077062;-8.9076283071190119;-8.9076283071190119;-10.228154513053596;-10.228154513053596;-10.228154513053596;-10.228154513053596;-10.228154513053596;-10.228154513053596;-10.747893488034606;-10.747893488034606;-10.747893488034606;-10.747893488034606;-11.005469451658428;-11.005469451658428;-11.005469451658428;-11.005469451658428]  xmax=[2.554547494451981;2.554547494451981;2.554547494451981;2.554547494451981;2.554547494451981;3.2832369712996297;3.2832369712996297;3.2832369712996297;4.0846229008166119;4.0878605725592934;4.9442778149386868;4.9442778149386868;4.9442778149386868;4.9442778149386868;4.9442778149386868;4.9442778149386868;4.9442778149386868;4.9442778149386868;4.9442778149386868;5.375724682235159;6.5858961467747577;6.5858961467747577;6.5858961467747577;6.5858961467747577;6.5858961467747577;6.5858961467747577;6.5858961467747577;6.5858961467747577;6.5858961467747577;7.8478635863866657;8.2404385135741904;8.2404385135741904;8.2404385135741904;8.2404385135741904;8.2404385135741904;8.9900587922893465;8.9900587922893465;8.9900587922893465;8.9900587922893465;9.9209288158454001;10.370046979689505;10.370046979689505;10.370046979689505;10.370046979689505;10.621967219631188;10.621967219631188;10.621967219631188;10.621967219631188;10.621967219631188;2.6554660173133016;3.688507386483252;3.688507386483252;3.688507386483252;3.688507386483252;3.688507386483252;3.688507386483252;3.688507386483252;3.688507386483252;4.4658235004171729;4.4658235004171729;4.4658235004171729;4.4658235004171729;4.4658235004171729;4.4658235004171729;4.4658235004171729;5.2941223829984665;5.2941223829984665;5.2941223829984665;6.1314987763762474;6.3656010450795293;6.3656010450795293;6.3656010450795293;6.3656010450795293;6.3656010450795293;6.3656010450795293;7.1818872513249516;7.1818872513249516;7.1818872513249516;8.2533658212050796;8.2533658212050796;8.2533658212050796;8.2533658212050796;8.2533658212050796;8.2533658212050796;8.2533658212050796;8.6014474593102932;8.6014474593102932;8.6014474593102932;10.042097930796444;10.042097930796444;10.042097930796444;10.042097930796444;10.042097930796444;10.042097930796444;10.042097930796444;10.042097930796444;10.042097930796444;10.042097930796444]  ymin=-1  ymax=1
  removeconstantrows : neural/Processing Functions/removeconstantrows  inputSize=100  keep=[2 3 4 5 6 7 8 9 10 11 12 13 14 15 16 17 18 19 20 21 22 23 24 25 26 27 28 29 30 31 32 33 34 35 36 37 38 39 40 41 42 43 44 45 46 47 48 49 50 52 53 54 55 56 57 58 59 60 61 62 63 64 65 66 67 68 69 70 71 72 73 74 75 76 77 78 79 80 81 82 83 84 85 86 87 88 89 90 91 92 93 94 95 96 97 98 99 100]
  p : Outport  PortDimensions=98
      mask Display: e = 0.06;c1 = [120 230 180]/255;c2 = ([120 230 180]+0)/(256+128);c3 = ([120 230 180]+128)/(256+128);patch([0 1 1 0],[0 0 1 1],c1);patch([0 1 1 1-e 1-e 0+e],[0 0 1 1-e 0+e 0+e],c2);patch([0 0 1 1-e 0+e 0+e],[0 1 1 1-e 1-e 0+e],c3);plot([0 1 1 0 0],[0 0 1 1 0]);
  wires:
  x/1 -> removeconstantrows/1
  removeconstantrows/1 -> mapminmax/1
  mapminmax/1 -> p/1

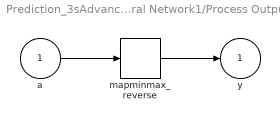
== system Prediction_3sAdvance_2output/Function Fitting Neural Network1/Process Output 1 ==
  a : Inport  PortDimensions=2
      mask Display: e = 0.06;c1 = [120 230 180]/255;c2 = ([120 230 180]+0)/(256+128);c3 = ([120 230 180]+128)/(256+128);patch([0 1 1 0],[0 0 1 1],c1);patch([0 1 1 1-e 1-e 0+e],[0 0 1 1-e 0+e 0+e],c2);patch([0 0 1 1-e 0+e 0+e],[0 1 1 1-e 1-e 0+e],c3);plot([0 1 1 0 0],[0 0 1 1 0]);
  mapminmax_reverse : neural/Processing Functions/mapminmax_reverse  xmin=[-7.8478635863866657;-8.2533658212050796]  xmax=[7.8414806934306398;8.7490837695077062]  ymin=-1  ymax=1
  y : Outport  PortDimensions=2
      mask Display: e = 0.06;c1 = [120 230 180]/255;c2 = ([120 230 180]+0)/(256+128);c3 = ([120 230 180]+128)/(256+128);patch([0 1 1 0],[0 0 1 1],c1);patch([0 1 1 1-e 1-e 0+e],[0 0 1 1-e 0+e 0+e],c2);patch([0 0 1 1-e 0+e 0+e],[0 1 1 1-e 1-e 0+e],c3);plot([0 1 1 0 0],[0 0 1 1 0]);
  wires:
  a/1 -> mapminmax_reverse/1
  mapminmax_reverse/1 -> y/1

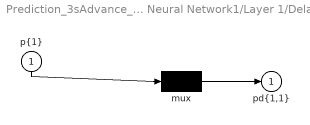
== system Prediction_3sAdvance_2output/Function Fitting Neural Network1/Layer 1/Delays 1 ==
  "p{1}" : Inport  PortDimensions=98
      mask Display: e = 0.06;c1 = [120 230 180]/255;c2 = ([120 230 180]+0)/(256+128);c3 = ([120 230 180]+128)/(256+128);patch([0 1 1 0],[0 0 1 1],c1);patch([0 1 1 1-e 1-e 0+e],[0 0 1 1-e 0+e 0+e],c2);patch([0 0 1 1-e 0+e 0+e],[0 1 1 1-e 1-e 0+e],c3);plot([0 1 1 0 0],[0 0 1 1 0]);
  mux : Mux  Inputs=1
      mask Display: e = 0.06;c1 = [120 150 230]/255;c2 = ([120 150 230]+0)/383;c3 = ([120 150 230]+128)/383;patch([0 1 1 0],[0 0 1 1],c1);patch([0 1 1 1-e 1-e 0+e],[0 0 1 1-e 0+e 0+e],c2);patch([0 0 1 1-e 0+e 0+e],[0 1 1 1-e 1-e 0+e],c3);plot([0 1 1 0 0],[0 0 1 1 0]);disp('Mux')
  "pd{1,1}" : Outport
      mask Display: e = 0.06;c1 = [120 230 180]/255;c2 = ([120 230 180]+0)/(256+128);c3 = ([120 230 180]+128)/(256+128);patch([0 1 1 0],[0 0 1 1],c1);patch([0 1 1 1-e 1-e 0+e],[0 0 1 1-e 0+e 0+e],c2);patch([0 0 1 1-e 0+e 0+e],[0 1 1 1-e 1-e 0+e],c3);plot([0 1 1 0 0],[0 0 1 1 0]);
  wires:
  "p{1}"/1 -> mux/1
  mux/1 -> "pd{1,1}"/1
